simulink model "IO424_Resolver_signal_gen"  (R2024b)
settings: Solver=FixedStepDiscrete  StartTime=0.0  StopTime=0.15  FixedStep=1e-6  RelTol=1e-3
settings Model: Creator=aleandro.vegni  LastModifiedBy=nathan.gyger

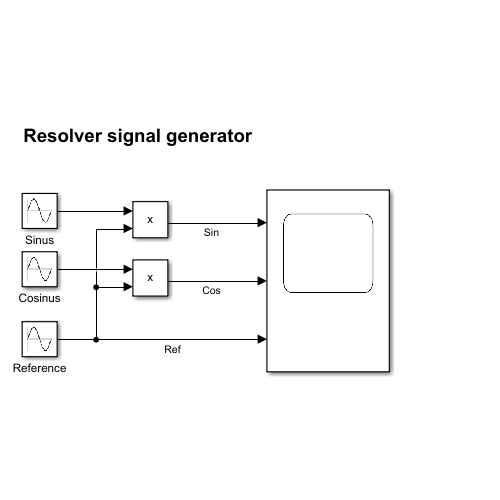
[thumbnail: Simulink's stored preview of the top-level diagram]
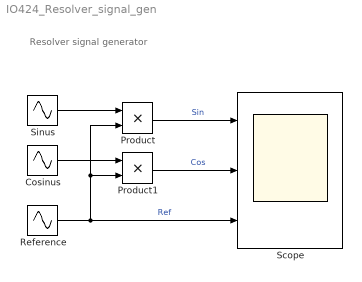
== system IO424_Resolver_signal_gen ==
  note: Resolver signal generator
  Cosinus : Sin  Amplitude=0.5  Frequency=2*pi*10  Phase=pi/2  SampleTime=0
  Product : Product
  Product1 : Product
  Reference : Sin  Amplitude=4*sqrt(2)  Frequency=2*pi*1e3  SampleTime=0
  Scope : Scope  NumInputPorts=3
  Sinus : Sin  Amplitude=0.5  Frequency=2*pi*10  SampleTime=0
  wires:
  Sinus/1 -> Product/1
  Reference/1 -> Product/2, Product1/2, Scope/3  "Ref"
  Product/1 -> Scope/1  "Sin"
  Cosinus/1 -> Product1/1
  Product1/1 -> Scope/2  "Cos"
